simulink model "simulation_reduced_system_with_fault"  (R2021b)
settings: Solver=ode23t  StartTime=0.0  StopTime=0.2  MaxStep=5e-5  RelTol=1e-3  AbsTol=1e-2
undefined symbols (not defined in the file): A, A_approx_bisimulation, B, B_approx_bisimulation, C, C_approx_bisimulation, D, D_approx_bisimulation, initial_states, initial_states_approx_bisimulation
libraries: spsThreePhaseFaultLib x4, spsThreePhaseProgrammableVoltageSourceLib x2, spsThreePhaseVIMeasurementLib x2, spsGroundLib x2, spspowerguiLib x1
settings Model: Creator=The MathWorks, Inc.  LastModifiedBy=amparogonzalezcastano
settings SolverCC: AutoScaleAbsTol=off  AlgebraicLoopSolver=TrustRegion
settings DataIOCC: Decimation=10  SaveFinalState=on  SaveFormat=Array  SaveOutput=off  ReturnWorkspaceOutputs=off  SignalLoggingName=sigsOut
settings OptimizationCC: BlockReduction=off  BooleanDataType=off  ExpressionDepthLimit=2147483647  InitFltsAndDblsToZero=on  LifeSpan=inf
settings DebuggingCC: UnderspecifiedInitializationDetection=Classic  MergeDetectMultiDrivingBlocksExec=none  CheckExecutionContextPreStartOutputMsg=on  SignalResolutionControl=TryResolveAllWithWarning  MultiTaskDSMMsg=warning  MultiTaskCondExecSysMsg=none  SigSpecEnsureSampleTimeMsg=none  FcnCallInpInsideContextMsg=warning  UnconnectedInputMsg=none  UnconnectedOutputMsg=none  StateNameClashWarn=warning  SFUnexpectedBacktrackingDiag=warning  SFNoUnconditionalDefaultTransitionDiag=warning  SFExecutionAtInitializationDiag=none  SFMachineParentedDataDiag=warning  ArithmeticOperatorsInVariantConditions=warning
settings HardwareCC: ProdBitPerPointer=32  ProdBitPerSizeT=32  ProdBitPerPtrDiffT=32  ProdLargestAtomicFloat=None  ProdIntDivRoundTo=Undefined  ProdEndianess=Unspecified  ProdWordSize=32  ProdHWDeviceType=Specified  TargetUnknown=on
settings ModelReferenceCC: PropagateSignalLabelsOutOfModel=off
settings SFSimCC: SimUseLocalCustomCode=off  CustomCodeUndefinedFunction=UseInterfaceOnly
settings RTWCC: RTWUseLocalCustomCode=off
settings CodeAppCC: StateflowObjectComments=on
settings GRTTargetCC: TargetLangStandard=C89/C90 (ANSI)  CombineOutputUpdateFcns=off  GRTInterface=on
settings ConfigComp: CovMetricSettings=dw  CovSaveCumulativeToWorkspaceVar=on  CovSaveSingleToWorkspaceVar=on  CovExternalEMLEnable=off  CovSFcnEnable=off
settings SimscapeCC: SimscapeNormalizeSystem=off

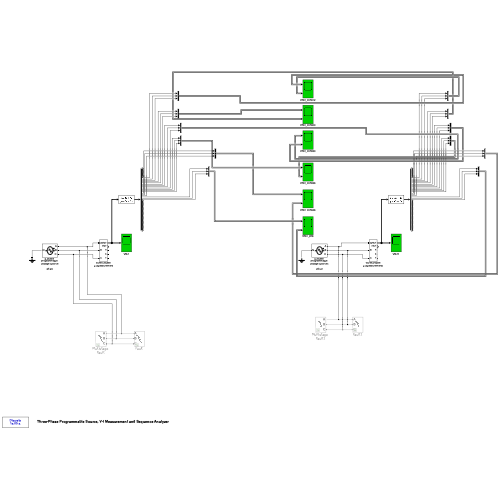
[thumbnail: Simulink's stored preview of the top-level diagram]
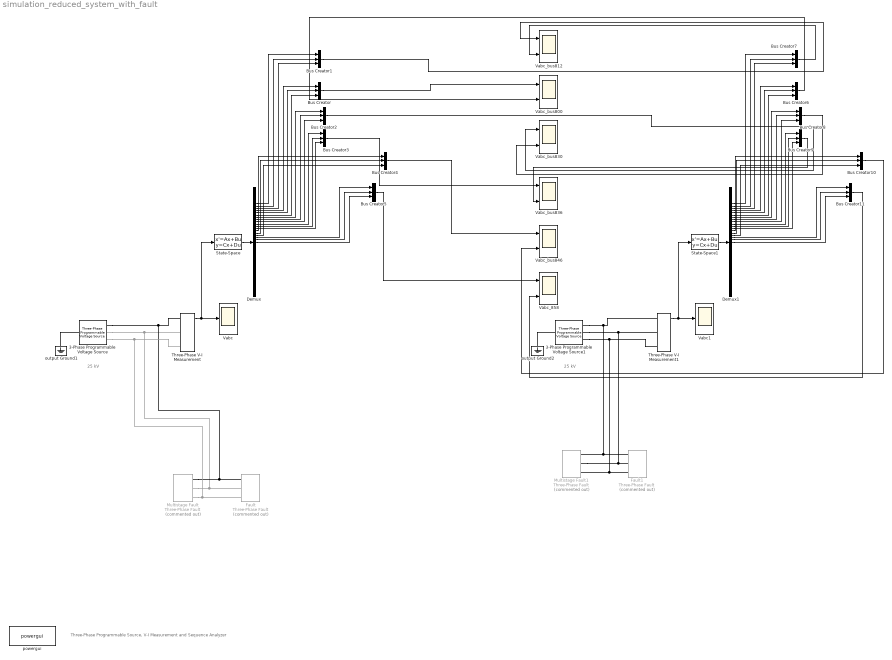
== system simulation_reduced_system_with_fault ==
  note: Three-Phase Programmable Source, V-I Measurement and Sequence Analyzer
  note: 25 kV
  note: 25 kV
  3-Phase Programmable Voltage Source : spsThreePhaseProgrammableVoltageSourceLib/Three-Phase Programmable Voltage Source  PositiveSequence="[25e3 0  60]"  VariationEntity=Amplitude  VariationType=Step  VariationTypeAlt=Step  VariationStep=0.5  VariationRate=10  VariationMagnitude=0.3  VariationFrequency=2  VariationTiming=[0 0.5]  VariationPhaseA=off  Amplitudes=[1 0.8 1.2 1.0]  TimeValues=[0 0.1 0.15 0.2]  HarmonicGeneration=off  HarmonicA=[5 0.08 -45 2]  HarmonicB=[2 0 0 2]  Timing="[0.1  1]"  BusType=swing  Pref=0  Qref=0  Qmin=-inf  Qmax=inf
  3-Phase Programmable Voltage Source1 : spsThreePhaseProgrammableVoltageSourceLib/Three-Phase Programmable Voltage Source  PositiveSequence="[25e3 0  60]"  VariationEntity=Amplitude  VariationType=Step  VariationTypeAlt=Step  VariationStep=0.5  VariationRate=10  VariationMagnitude=0.3  VariationFrequency=2  VariationTiming=[0 0.5]  VariationPhaseA=off  Amplitudes=[1 0.8 1.2 1.0]  TimeValues=[0 0.1 0.15 0.2]  HarmonicGeneration=off  HarmonicA=[5 0.08 -45 2]  HarmonicB=[2 0 0 2]  Timing="[0.1  1]"  BusType=swing  Pref=0  Qref=0  Qmin=-inf  Qmax=inf
  Bus Creator{,1..11} (12 alike) : BusCreator  Inputs=3
  Demux : Demux  Outputs=49
  Demux1 : Demux  Outputs=49
  Fault : spsThreePhaseFaultLib/Three-Phase Fault  Commented=on  InitialStates=0  FaultA=on  FaultB=on  FaultC=on  GroundFault=on  SwitchTimes=[ 0.01 0.05 0.08 0.1 0.15]  External=off  SwitchStatus=NaN  FaultResistance=1  GroundResistance=0.01  SnubberResistance=1e6  SnubberCapacitance=inf  Measurements=None
  Fault1 : spsThreePhaseFaultLib/Three-Phase Fault  Commented=on  InitialStates=0  FaultA=on  FaultB=on  FaultC=on  GroundFault=on  SwitchTimes=[ 0.01 0.05 0.08 0.1 0.15]  External=off  SwitchStatus=NaN  FaultResistance=1  GroundResistance=0.01  SnubberResistance=1e6  SnubberCapacitance=inf  Measurements=None
  Multistage Fault : spsThreePhaseFaultLib/Three-Phase Fault  Commented=on  InitialStates=0  FaultA=on  FaultB=on  FaultC=on  GroundFault=on  SwitchTimes=[ 0.02 0.05 0.08 0.15]  External=off  SwitchStatus=NaN  FaultResistance=0.1  GroundResistance=0.01  SnubberResistance=1e6  SnubberCapacitance=inf  Measurements=None
  Multistage Fault1 : spsThreePhaseFaultLib/Three-Phase Fault  Commented=on  InitialStates=0  FaultA=on  FaultB=on  FaultC=on  GroundFault=on  SwitchTimes=[ 0.02 0.05 0.08 0.15]  External=off  SwitchStatus=NaN  FaultResistance=0.1  GroundResistance=0.01  SnubberResistance=1e6  SnubberCapacitance=inf  Measurements=None
  State-Space : StateSpace  A=A  B=B  C=C  D=D  InitialCondition=initial_states  AllowTunableDMatrix=on
  State-Space1 : StateSpace  A=A_approx_bisimulation  B=B_approx_bisimulation  C=C_approx_bisimulation  D=D_approx_bisimulation  InitialCondition=initial_states_approx_bisimulation  AllowTunableDMatrix=on
  Three-Phase V-I Measurement : spsThreePhaseVIMeasurementLib/Three-Phase V-I Measurement  VoltageMeasurement=phase-to-ground  SetLabelV=off  LabelV=V1  Vpu=off  VpuLL=off  CurrentMeasurement=yes  SetLabelI=off  LabelI=I1  Ipu=off  Pbase=100e6  Vbase=25e3  OutputType=Magnitude  PhasorSimulation=off  PSBequivalent=0
  Three-Phase V-I Measurement1 : spsThreePhaseVIMeasurementLib/Three-Phase V-I Measurement  VoltageMeasurement=phase-to-ground  SetLabelV=off  LabelV=V1  Vpu=off  VpuLL=off  CurrentMeasurement=yes  SetLabelI=off  LabelI=I1  Ipu=off  Pbase=100e6  Vbase=25e3  OutputType=Magnitude  PhasorSimulation=off  PSBequivalent=0
  Vabc : Scope
  Vabc1 : Scope
  Vabc_858 : Scope  NumInputPorts=2
  Vabc_bus{800,812,830,836,846} (5 alike) : Scope  NumInputPorts=2
  output Ground1 : spsGroundLib/Ground  LConnTagsString=a
  output Ground2 : spsGroundLib/Ground  LConnTagsString=a
  powergui : spspowerguiLib/powergui  Priority=2  SimulationMode=Discrete  SampleTime=10e-6  frequency=60  Iterations=50  frequencyindice=60  Pbase=100e6  ErrMax=1e-4  UnitsV=kV  UnitsW=MW  buscounter=0  FunctionMessages=off  echomessages=off  EnableUseOfTLC=off  CurrentSourceSwitches=off  DisableSnubberDevices=off  DisableRonSwitches=off  DisableVfSwitches=off  DisplayEquations=off  AutomaticDiscreteSolvers=off  SolverType=Tustin/Backward Euler (TBE)  Interpol=off  ExternalGateDelay=off  methode=off  Ts=0  x0status=blocks  SPID=off  SwTol=0  HookPort=off  NonlinearTolerance=1e-1  nMaxIteration=100  ContinueOnMaxIteration=off  RestoreLinks=warning  ResistiveCurrentMeasurement=off  Frange=[0:2:500]  Ylog=off  Xlog=off  ShowGrid=off  save=off  variable=ZData  structure=0  ZoomFFT=on  StartTime=0.0  cycles=1  DisplayStyle=off  fundamental=60  FreqAxis=off  MaxFrequency=1000  frequencyindicesteady=1  RmsSteady=1  display=off
  wires:
  Three-Phase V-I Measurement/1 -> Vabc/1, State-Space/1
  State-Space/1 -> Demux/1
  Demux/8 -> Bus Creator1/1
  Demux/9 -> Bus Creator1/2
  Demux/10 -> Bus Creator1/3
  Demux/11 -> Bus Creator/1
  Demux/12 -> Bus Creator/2
  Demux/13 -> Bus Creator/3
  Demux/14 -> Bus Creator2/1
  Demux/15 -> Bus Creator2/2
  Demux/16 -> Bus Creator2/3
  Demux/17 -> Bus Creator3/1
  Demux/18 -> Bus Creator3/2
  Demux/19 -> Bus Creator3/3
  Demux/20 -> Bus Creator4/1
  Demux/21 -> Bus Creator4/2
  Demux/22 -> Bus Creator4/3
  Bus Creator/1 -> Vabc_bus800/1
  Bus Creator1/1 -> Vabc_bus812/1
  Bus Creator2/1 -> Vabc_bus830/1
  Bus Creator3/1 -> Vabc_bus836/1
  Bus Creator4/1 -> Vabc_bus846/1
  Bus Creator5/1 -> Vabc_858/1
  Demux/23 -> Bus Creator5/1
  Demux/24 -> Bus Creator5/2
  Demux/25 -> Bus Creator5/3
  Demux1/12 -> Bus Creator6/2
  Bus Creator11/1 -> Vabc_858/2
  Demux1/20 -> Bus Creator10/1
  Bus Creator8/1 -> Vabc_bus830/2
  State-Space1/1 -> Demux1/1
  Demux1/18 -> Bus Creator9/2
  Demux1/23 -> Bus Creator11/1
  Bus Creator7/1 -> Vabc_bus812/2
  Three-Phase V-I Measurement1/1 -> Vabc1/1, State-Space1/1
  Demux1/13 -> Bus Creator6/3
  Demux1/15 -> Bus Creator8/2
  Demux1/9 -> Bus Creator7/2
  Demux1/21 -> Bus Creator10/2
  Demux1/8 -> Bus Creator7/1
  Bus Creator10/1 -> Vabc_bus846/2
  Demux1/11 -> Bus Creator6/1
  Demux1/16 -> Bus Creator8/3
  Demux1/25 -> Bus Creator11/3
  Demux1/19 -> Bus Creator9/3
  Demux1/17 -> Bus Creator9/1
  Demux1/14 -> Bus Creator8/1
  Demux1/22 -> Bus Creator10/3
  Bus Creator9/1 -> Vabc_bus836/2
  Bus Creator6/1 -> Vabc_bus800/2
  Demux1/10 -> Bus Creator7/3
  Demux1/24 -> Bus Creator11/2
  connections:
  output Ground1/LConn1 -- 3-Phase Programmable Voltage Source/LConn1
  Multistage Fault/LConn2 -- Fault/LConn2 -- 3-Phase Programmable Voltage Source/RConn2 -- Three-Phase V-I Measurement/LConn2
  3-Phase Programmable Voltage Source/RConn1 -- Fault/LConn1 -- Multistage Fault/LConn1 -- Three-Phase V-I Measurement/LConn1
  output Ground2/LConn1 -- 3-Phase Programmable Voltage Source1/LConn1
  3-Phase Programmable Voltage Source1/RConn2 -- Multistage Fault1/LConn2 -- Fault1/LConn2 -- Three-Phase V-I Measurement1/LConn2
  Fault/LConn3 -- Multistage Fault/LConn3 -- 3-Phase Programmable Voltage Source/RConn3 -- Three-Phase V-I Measurement/LConn3
  3-Phase Programmable Voltage Source1/RConn1 -- Fault1/LConn1 -- Multistage Fault1/LConn1 -- Three-Phase V-I Measurement1/LConn1
  3-Phase Programmable Voltage Source1/RConn3 -- Fault1/LConn3 -- Multistage Fault1/LConn3 -- Three-Phase V-I Measurement1/LConn3
